simulink model "ACS_LONG_AP_MODAL_CL"  (R2022b)
settings: Solver=VariableStepAuto  StartTime=0.0  StopTime=500  RelTol=1e-3
undefined symbols (not defined in the file): H_long_1, K_long1_y
libraries: cstblocks x1
settings Model: Creator=bendr  LastModifiedBy=bendr

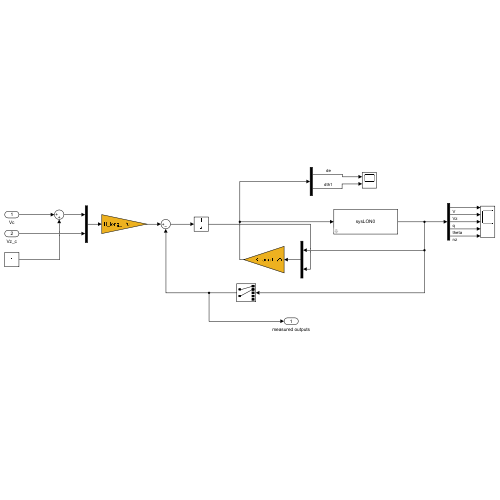
[thumbnail: Simulink's stored preview of the top-level diagram]
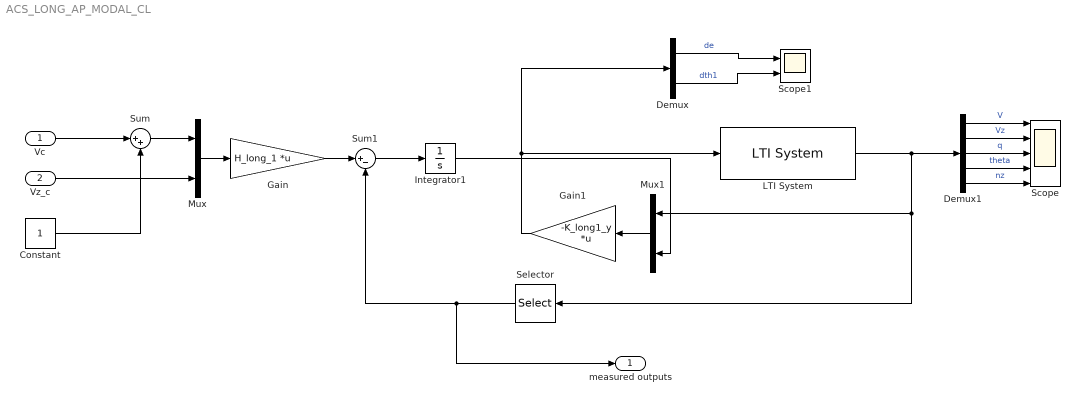
== system ACS_LONG_AP_MODAL_CL ==
  Vc : Inport
  Vz_c : Inport  Port=2
  Constant : Constant
  Demux : Demux  Outputs=2
  Demux1 : Demux  Outputs=5
  Gain : Gain  Gain=H_long_1  Multiplication=Matrix(K*u)
  Gain1 : Gain  Gain=-K_long1_y  Multiplication=Matrix(K*u)
  Integrator1 : Integrator
  LTI System : cstblocks/LTI System  sys=sysLON0  IC=[]
  Mux : Mux  Inputs=2
  Mux1 : Mux  Inputs=2
  Scope : Scope  NumInputPorts=5
  Scope1 : Scope  NumInputPorts=2
  Selector : Selector  InputPortWidth=5  IndexOptions=Index vector (dialog)  Indices=[1 2]  OutputSizes=1
  Sum : Sum  Inputs=|++
  Sum1 : Sum  Inputs=|+-
  measured outputs : Outport
  wires:
  LTI System/1 -> Mux1/1, Selector/1, Demux1/1
  Sum1/1 -> Integrator1/1
  Vz_c/1 -> Mux/2
  Mux/1 -> Gain/1
  Gain/1 -> Sum1/1
  Selector/1 -> Sum1/2, measured outputs/1
  Integrator1/1 -> Mux1/2
  Mux1/1 -> Gain1/1
  Vc/1 -> Sum/1
  Sum/1 -> Mux/1
  Constant/1 -> Sum/2
  Demux/1 -> Scope1/1  "de"
  Demux/2 -> Scope1/2  "dth1"
  Gain1/1 -> LTI System/1, Demux/1
  Demux1/1 -> Scope/1  "V"
  Demux1/2 -> Scope/2  "Vz"
  Demux1/3 -> Scope/3  "q"
  Demux1/4 -> Scope/4  "theta"
  Demux1/5 -> Scope/5  "nz"
